simulink library "KL_HignVoltageSimuCtl"  (Simulink 7.8)
settings: Solver=ode45  StartTime=0.0  StopTime=10.0  RelTol=1e-3
settings Model: Creator=Administrator  LastModifiedBy=KLJS195

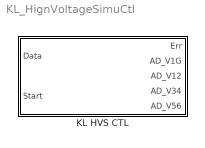
== system KL_HignVoltageSimuCtl ==
  KL HVS CTL : Subsystem  mask(KL High Voltage Simulation Model){CtlId=0, rev0=TCP/IP, DestIp=[192 168 2 240], DestPort=2040, rev1=1, rev2=1, rev3=0, rev4=0}
      mask prompts: CtlId "Control ID"; rev0 "TCP/IP Client or SoftingCanPci"; DestIp "Dest IP"; rev1 "Can Card Index"; rev2 "Card Channel"
      mask StyleString: edit,popup(TCP/IP|SoftingCanPci),edit,edit,edit,popup(1|2),edit,edit
      mask CallbackString:
      | |bco = get_param(gcb,'rev0');
      | if(strcmp(bco,'TCP/IP')),
      |     set_param(gcb,'MaskVisibilities',{'on';'on';'on';'on';'off';'off';'off';'off'}),
      | else
      |     set_param(gcb,'MaskVisibilities',{'on';'on';'off';'off';'on';'on';'off';'off'}),
      | end||||||
      mask Display: disp (sprintf ('Control ID: %d', CtlId))

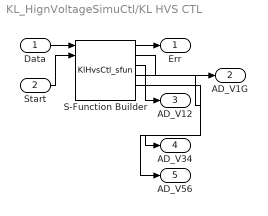
== system KL_HignVoltageSimuCtl/KL HVS CTL ==
  Data : Inport
  Start : Inport  Port=2
  S-Function Builder : S-Function  InitFcn=try, set_param(gcb,'FunctionName','KlHvsCtl_sfun'), end  FunctionName=KlHvsCtl_sfun  Parameters=CtlId,DestIp,DestPort,rev0,rev1,rev2,rev3,rev4  WizardData=DataTag0  EnableBusSupport=off  mask(S-Function Builder){}
      mask help: Simulink:masks:SFunctionBuilder_MD
      mask init:
      | val = [[.9  0.75 0.75 1 1 .9 .9 1]',[1 1 0.75 0.75 .9 .9 1 .9]'];try , sys = get_param(gcb,'SfunBuilderFcnName');if isempty(sys), sys = get_param(gcb,'FunctionName'); end,catch, sys = get_param(gcb,'FunctionName'); end
      settings: CopyFcn=set_param(gcbh,'LinkStatus','none')  PreSaveFcn=try, set_param(gcb,'FunctionName','KlHvsCtl_sfun'), end  OpenFcn=sfunctionwizard(gcbh)
      mask Display: plot(val(:,1),val(:,2)),disp(sys), port_label('input',1,'u0'), port_label('input',2,'u1'), port_label('input',3,'u2'), port_label('input',4,'u3'), port_label('input',5,'u4'), port_label('input',6,'u5'), port_label('output',1,'y0'), port_label('output',2,'y1'), port_label('output',3,'y2'), port_label('output',4,'y3'), port_label('output',5,'y4'), port_label('output',6,'y5')
  Err : Outport
  AD_V1G : Outport  Port=2
  AD_V12 : Outport  Port=3
  AD_V34 : Outport  Port=4
  AD_V56 : Outport  Port=5
  wires:
  Start/1 -> S-Function Builder/2
  Data/1 -> S-Function Builder/1
  S-Function Builder/1 -> Err/1
  S-Function Builder/2 -> AD_V1G/1
  S-Function Builder/3 -> AD_V12/1
  S-Function Builder/4 -> AD_V34/1
  S-Function Builder/5 -> AD_V56/1
